simulink model "IAPF"  (R2025b)
settings: Solver=ode4  StartTime=0.0  StopTime=200  FixedStep=0.01  RelTol=1e-3
values from neighbouring files (symbols this model uses):
  A = zeros(num_agents, num_agents)    [init.m]
  D_des = zeros(num_agents, num_agents)    [init.m]
  k_a = 100    [init.m]
  k_d = 5    [init.m]
  k_e = 50    [init.m]
  k_r = 50    [init.m]
  k_t = 0.1    [init.m]
  n_goal = 2    [init.m]
  obs_center = [50; 50; 50]    [init.m]
  obs_rho0 = 25    [init.m]
  p0_all = repmat(q_start, 1, num_agents) + delta    [init.m]
  q_target = [100; 100; 100]    [init.m]
  v0_all = zeros(3, num_agents)    [init.m]
settings Model: Creator=ZhuanZ（无密码）  LastModifiedBy=ZhuanZ（无密码）

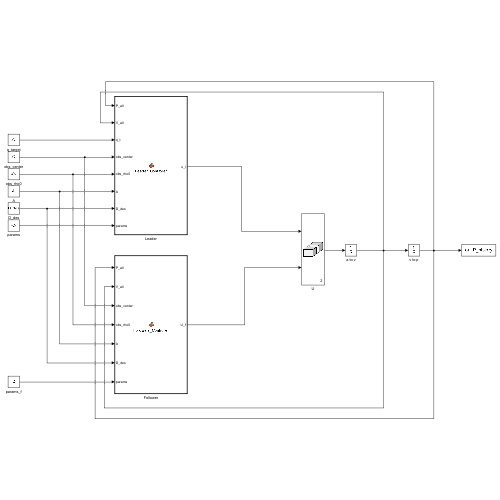
[thumbnail: Simulink's stored preview of the top-level diagram]
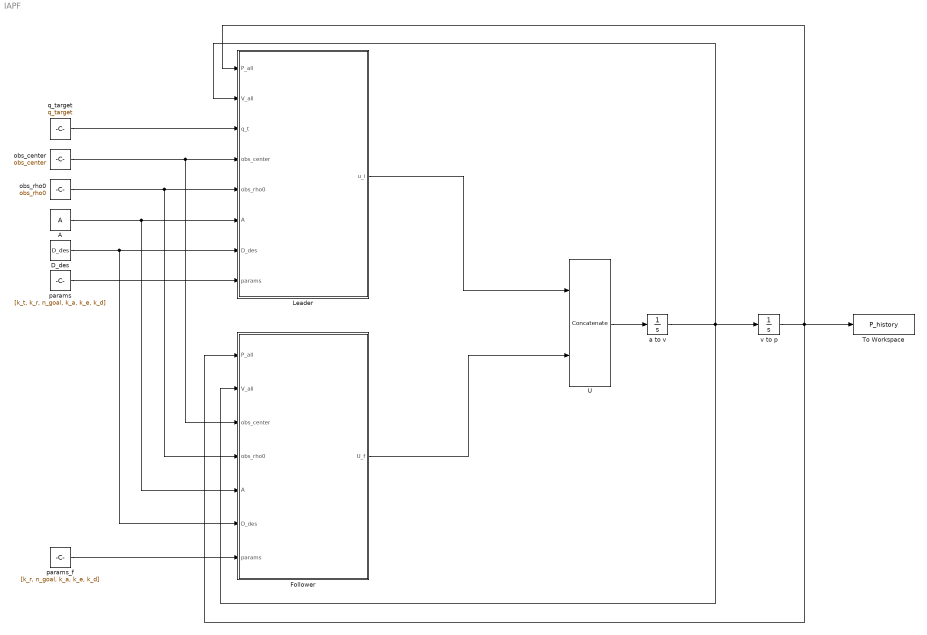
== system IAPF ==
  A : Constant  Value=A
  D_des : Constant  Value=D_des
  Follower : MATLAB Function  TreatAsAtomicUnit=on
  Leader : MATLAB Function  TreatAsAtomicUnit=on
  To Workspace : ToWorkspace  VariableName=P_history  SampleTime=-1
  U : Concatenate  Mode=Multidimensional array  ConcatenateDimension=2
  a to v : Integrator  InitialCondition=v0_all
  obs_center : Constant  Value=obs_center
  obs_rho0 : Constant  Value=obs_rho0
  params : Constant  Value=[k_t, k_r, n_goal, k_a, k_e, k_d]
  params_f : Constant  Value=[k_r, n_goal, k_a, k_e, k_d]
  q_target : Constant  Value=q_target
  v to p : Integrator  InitialCondition=p0_all
  wires:
  params/1 -> Leader/8(params)
  A/1 -> Leader/6(A), Follower/5(A)
  D_des/1 -> Leader/7(D_des), Follower/6(D_des)
  obs_center/1 -> Leader/4(obs_center), Follower/3(obs_center)
  obs_rho0/1 -> Leader/5(obs_rho0), Follower/4(obs_rho0)
  q_target/1 -> Leader/3(q_t)
  Leader/1(u_i) -> U/1
  Follower/1(U_f) -> U/2
  U/1 -> a to v/1
  a to v/1 -> Leader/2(V_all), Follower/2(V_all), v to p/1
  v to p/1 -> To Workspace/1, Leader/1(P_all), Follower/1(P_all)
  params_f/1 -> Follower/7(params)

== matlab function IAPF/Follower ==
  data: P_all input; U_f output; V_all input; obs_center input; obs_rho0 input; A input; D_des input; params input
function U_f = Followers_Controller(P_all, V_all, obs_center, obs_rho0, A, D_des, params)
    % =====================================================================
    % 输入说明：
    % P_all: 3xN 矩阵，所有无人机位置 (第1列为Leader)
    % V_all: 3xN 矩阵，所有无人机速度 (用于给每架跟随者分配阻尼)
    % obs_center, obs_rho0, A, D_des 同 Leader 模块
    % params: 1x5 数组 [k_r, n_goal, k_a, k_e, k_d] (去掉了 k_t)
    %
    % 输出说明：
    % U_f: 3 x (N-1) 矩阵，依次代表 2~N 号跟随者的合力 (加速度)
    % =====================================================================
    
    % 解析控制参数
    k_r     = params(1);
    n_goal  = params(2);
    k_a     = params(3);
    k_e     = params(4);
    k_d     = params(5);
    
    num_agents = size(P_all, 2);
    U_f = zeros(3, num_agents - 1); % 初始化输出矩阵
    p_leader = P_all(:, 1);         % 提取领航者位置，作为虚拟目标
    
    epsilon = 1e-6; 

    % =====================================================================
    % 核心：For 循环遍历每一个跟随者 (从 2 到 N)
    % =====================================================================
    for i = 2:num_agents
        p_i = P_all(:, i);
        v_i = V_all(:, i);
        
        %% 1. 障碍物斥力 (F_r) - 使用到 Leader 的距离作为 GNRON 衰减因子
        F_r = zeros(3, 1);
        rho_o = norm(p_i - obs_center);
        n_op = (p_i - obs_center) / (rho_o + epsilon); 
        
        if rho_o <= obs_rho0
            % 计算到 Leader 的距离作为虚拟目标距离 rho_g
            rho_g = norm(p_i - p_leader);
            n_pg = (p_i - p_leader) / (rho_g + epsilon);
            
            % F_rep1: 推离障碍物
            term1 = k_r * (1/rho_o - 1/obs_rho0) * (rho_g^n_goal) / (rho_o^2);
            F_rep1 = term1 * n_op;
            
            % F_rep2: 拉向虚拟目标 (Leader方向)
            term2 = (n_goal / 2) * k_r * (1/rho_o - 1/obs_rho0)^2 * (rho_g^(n_goal-1));
            F_rep2 = term2 * (-n_pg); 
            
            F_r = F_rep1 + F_rep2;
        end
        
        %% 2. 编队控制力 (F_form) - 遍历所有邻居
        F_form = zeros(3, 1);
        for j = 1:num_agents
            if A(i, j) == 1  % 查拓扑字典：j 是不是 i 的邻居？
                p_j = P_all(:, j);
                f_ij = norm(p_i - p_j);
                
                if f_ij > 0.1 % 防重合崩溃
                    d_des = D_des(i, j); % 查表获取两机间的期望距离
                    force_mag = -k_a * (1 - (d_des^2) / (f_ij^2));
                    F_ij = force_mag * ((p_i - p_j) / f_ij);
                    F_form = F_form + F_ij;
                end
            end
        end
        
        %% 3. 局部极小值旋转力 (F_e) - 使用 F_form 替代 F_a 进行死锁判定
        F_e = zeros(3, 1);
        if norm(F_form) > epsilon && norm(F_r) > epsilon
            % 判断编队拉力与障碍物斥力是否对冲
            cos_theta = dot(F_form, F_r) / (norm(F_form) * norm(F_r));
            
            if cos_theta <= -0.9
                e3 = [0; 0; 1]; 
                F_e = k_e * rho_o * cross(n_op, e3); 
            end
        end
        
        %% 4. 阻尼项与单机合力
        F_damp = -k_d * v_i;
        u_i = F_r + F_form + F_e + F_damp; % 注意：Follower 没有 F_a
        
        % 存入输出矩阵对应的列 (索引 i 从 2 开始，写入 U_f 的第 i-1 列)
        U_f(:, i-1) = u_i;
    end
end

== matlab function IAPF/Leader ==
  data: P_all input; u_i output; V_all input; q_t input; obs_center input; obs_rho0 input; A input; D_des input; params input
function u_i = Leader_Controller(P_all, V_all, q_t, obs_center, obs_rho0, A, D_des, params)
    % =====================================================================
    % 输入说明：
    % P_all: 3xN 矩阵，包含所有无人机的当前位置
    % v_i:   3x1 向量，Leader 当前的速度 (用于阻尼)
    % q_t:   3x1 向量，全局目标点位置
    % obs_center: 3x1 向量，障碍物中心坐标
    % obs_rho0: 标量，障碍物警戒半径
    % A:     NxN 邻接矩阵
    % D_des: NxN 期望距离矩阵
    % params: 1x6 数组，打包了所有增益系数 [k_t, k_r, n_goal, k_a, k_e, k_d]
    % =====================================================================
    
    % 解析控制参数
    k_t     = params(1);
    k_r     = params(2);
    n_goal  = params(3);
    k_a     = params(4);
    k_e     = params(5);
    k_d     = params(6);
    
    % Leader 永远是第 1 号节点
    p_i = P_all(:, 1);
    v_i = V_all(:, 1);
    num_agents = size(P_all, 2);
    
    % 防止距离为绝对的 0 导致除以 0 的 NaN 报错
    epsilon = 1e-6; 

    %% 1. 计算目标点引力 (F_a)
    rho_g = norm(p_i - q_t);
    n_pg = (p_i - q_t) / (rho_g + epsilon); % 指向目标的单位向量 (注意这里是 p-q_t)
    F_a = -k_t * rho_g * n_pg;              % 等价于 -k_t * (p_i - q_t)

    %% 2. 计算障碍物斥力 (F_r) - Ge & Cui 改进版
    F_r = zeros(3, 1);
    rho_o = norm(p_i - obs_center);
    n_op = (p_i - obs_center) / (rho_o + epsilon); % 从障碍物指向无人机的单位向量
    
    if rho_o <= obs_rho0
        % F_rep1: 推离障碍物的力 (方向 n_op)
        term1 = k_r * (1/rho_o - 1/obs_rho0) * (rho_g^n_goal) / (rho_o^2);
        F_rep1 = term1 * n_op;
        
        % F_rep2: 拉向目标的补丁力 (方向 -n_pg，即指向目标)
        term2 = (n_goal / 2) * k_r * (1/rho_o - 1/obs_rho0)^2 * (rho_g^(n_goal-1));
        F_rep2 = term2 * (-n_pg); 
        
        F_r = F_rep1 + F_rep2;
    end

    %% 3. 计算编队控制力 (F_form)
    F_form = zeros(3, 1);
    for j = 1:num_agents
        if A(1, j) == 1  % 查字典：如果节点 j 是我的邻居
            p_j = P_all(:, j);
            f_ij = norm(p_i - p_j);
            
            if f_ij > 0.1 % 加一个极小值保护，防止两机完全重合时 f_ij=0 导致崩溃
                d_des = D_des(1, j);
                % Pan 论文原版统一引斥力公式
                force_mag = -k_a * (1 - (d_des^2) / (f_ij^2));
                F_ij = force_mag * ((p_i - p_j) / f_ij);
                F_form = F_form + F_ij;
            end
        end
    end

    %% 4. 计算局部极小值旋转力 (F_e)
    F_e = zeros(3, 1);
    % 只有当同时受引力和斥力，且都不为 0 时，才可能陷入极小值
    if norm(F_a) > epsilon && norm(F_r) > epsilon
        % 计算引力与斥力的夹角余弦
        cos_theta = dot(F_a, F_r) / (norm(F_a) * norm(F_r));
        
        % 如果夹角接近 180 度 (互相抵消)
        if cos_theta <= -0.9
            e3 = [0; 0; 1]; % 旋转轴 (Z轴)
            % 产生切向旋转力
            F_e = k_e * rho_o * cross(n_op, e3); 
        end
    end

    %% 5. 阻尼项与合力输出
    F_damp = -k_d * v_i;
    
    % 最终输出给积分器的加速度 (合力)
    u_i = F_a + F_r + F_form + F_e + F_damp;

end
